simulink model "Battery_Model"  (R2017b)
settings: Solver=FixedStepAuto  StartTime=0.0  StopTime=1800  FixedStep=dt  RelTol=1e-3
PreLoadFcn:
  | Battery_Parameters
  | SOC_Curve
values from neighbouring files (symbols this model uses):
  bat_poly = p2    [Battery_Parameters.m]
  C1 = 6.9411e3 * N_Cell    (= 6941.1)    [Battery_Parameters.m]    (also in Module_Spec.m = zeros(1,Nb_cell_module))
  C2 = 8.8929 * N_Cell    (= 8.8929)    [Battery_Parameters.m]    (also in Module_Spec.m = zeros(1,Nb_cell_module))
  Capacity_max = 3113 * N_Cell    (= 3113)    [Battery_Parameters.m]    (also in Module_Spec.m = zeros(1,Nb_cell_module); SOC_Curve.m = SOC_data(end,1); Test_spec.m = Capacity_max_norm)
  R0 = 0.0715 / N_Cell    (= 0.0715)    [Battery_Parameters.m]    (also in Module_Spec.m = zeros(1,Nb_cell_module); Test_spec.m = R0_norm)
  R1 = 0.0227 / N_Cell    (= 0.0227)    [Battery_Parameters.m]    (also in Module_Spec.m = zeros(1,Nb_cell_module))
  R2 = 0.0103 / N_Cell    (= 0.0103)    [Battery_Parameters.m]    (also in Module_Spec.m = zeros(1,Nb_cell_module))
settings Model: Creator=christian-dsa  LastModifiedBy=christian
settings CodeAppCC: StateflowObjectComments=on
settings SimscapeCC: SimscapeNormalizeSystem=off

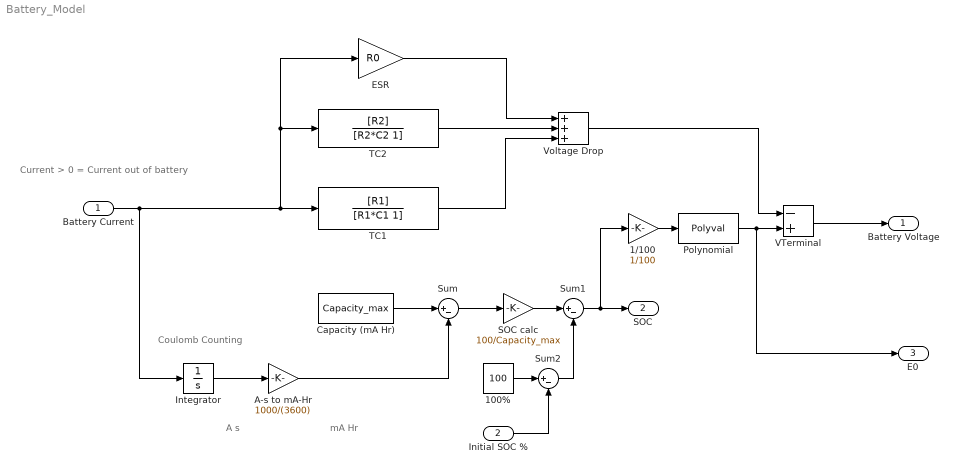
== system Battery_Model ==
  note: Current > 0 = Current out of battery
  note: A s
  note: mA Hr
  note: Coulomb Counting
  Battery Current : Inport
  Initial SOC % : Inport  Port=2
  1/100 : Gain  Gain=1/100
  100% : Constant  Value=100
  A-s to mA-Hr : Gain  Gain=1000/(3600)
  Capacity (mA Hr) : Constant  Value=Capacity_max
  ESR : Gain  Gain=R0
  Integrator : Integrator
  Polynomial : Polyval  Coefs=bat_poly
  SOC calc : Gain  Gain=100/Capacity_max
  Sum : Sum  Inputs=|+-
  Sum1 : Sum  Inputs=|+-
  Sum2 : Sum  Inputs=|+-
  TC1 : TransferFcn  Numerator=[R1]  Denominator=[R1*C1 1]
  TC2 : TransferFcn  Numerator=[R2]  Denominator=[R2*C2 1]
  VTerminal : Sum  Inputs=-+
  Voltage Drop : Sum  Inputs=+++
  Battery Voltage : Outport
  SOC : Outport  Port=2
  E0 : Outport  Port=3
  wires:
  Capacity (mA Hr)/1 -> Sum/1
  Sum/1 -> SOC calc/1
  A-s to mA-Hr/1 -> Sum/2
  Integrator/1 -> A-s to mA-Hr/1
  Polynomial/1 -> E0/1, VTerminal/2
  VTerminal/1 -> Battery Voltage/1
  TC1/1 -> Voltage Drop/3
  TC2/1 -> Voltage Drop/2
  ESR/1 -> Voltage Drop/1
  Voltage Drop/1 -> VTerminal/1
  Battery Current/1 -> Integrator/1, TC2/1, ESR/1, TC1/1
  SOC calc/1 -> Sum1/1
  Sum1/1 -> 1/100/1, SOC/1
  Initial SOC %/1 -> Sum2/2
  100%/1 -> Sum2/1
  Sum2/1 -> Sum1/2
  1/100/1 -> Polynomial/1
